simulink model "SMM_1"  (Simulink 8.1)
settings: Solver=ode45  StartTime=0.0  StopTime=20  MaxStep=1e-3  RelTol=1e-4  AbsTol=1e-6
InitFcn:
  | SMM_1_params
values from neighbouring files (symbols this model uses):
  alpha0 = 68  *pi/180    (= 1.18682389136)    [SMM_1_params.m]    (also in SMM_1_returnMap.m; SMM_1_roughTerrain.m)
  dx0 = 5    [SMM_1_params.m]    (also in SMM_1_returnMap.m = sqrt(2/m*(Esys-m*g*y0)))
  dy0 = 0    [SMM_1_params.m]    (also in SMM_1_returnMap.m; SMM_1_roughTerrain.m)
  g = 9.81    [SMM_1_params.m]    (also in SMM_1_returnMap.m; SMM_1_roughTerrain.m)
  k = 20000    [SMM_1_params.m]    (also in SMM_1_returnMap.m; SMM_1_roughTerrain.m)
  l0 = 1    [SMM_1_params.m]    (also in SMM_1_returnMap.m; SMM_1_roughTerrain.m)
  m = 70    [SMM_1_params.m]    (also in SMM_1_returnMap.m; SMM_1_roughTerrain.m)
  x0 = 0    [SMM_1_params.m]    (also in SMM_1_returnMap.m; SMM_1_roughTerrain.m)
  y0 = 1    [SMM_1_params.m]    (also in SMM_1_returnMap.m = v_y0(state))
libraries: simulink x1, simulink_extras x1
settings Model: Creator=hgeyer  LastModifiedBy=benshih
settings DebuggingCC: FcnCallInpInsideContextMsg=EnableAllAsWarning
settings GRTTargetCC: CombineOutputUpdateFcns=on  GRTInterface=off

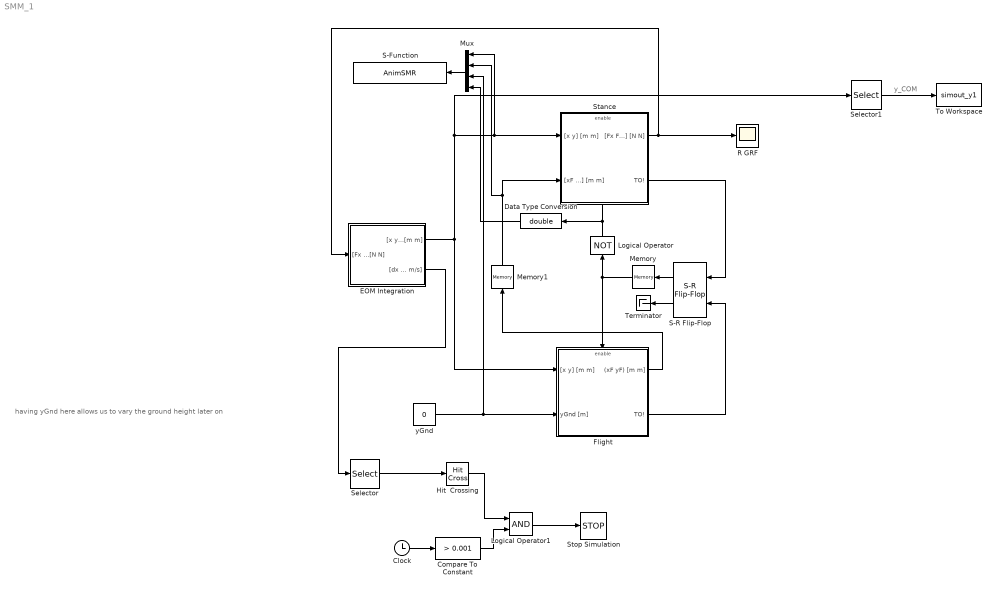
== system SMM_1 ==
  note: y_COM
  note: having yGnd here allows
      | us to vary the ground height later on
  Clock : Clock
  Compare To Constant : simulink/Logic and Bit Operations/Compare To Constant  relop=>  const=0.001  OutDataTypeStr=boolean
  Data Type Conversion : DataTypeConversion  OutDataTypeStr=double
  EOM Integration : Subsystem
  Flight : Subsystem
  Hit  Crossing : HitCross  HitCrossingDirection=falling
  Logical Operator : Logic  Operator=NOT  AllPortsSameDT=off  OutDataTypeStr=boolean
  Logical Operator1 : Logic  AllPortsSameDT=off  OutDataTypeStr=boolean
  Memory : Memory  X0=1
  Memory1 : Memory  X0=[0 0]
  Mux : Mux
  R GRF : Scope
  S-Function : S-Function  FunctionName=AnimSMR  Parameters=0.01  EnableBusSupport=off
  S-R Flip-Flop : simulink_extras/Flip Flops/S-R Flip-Flop  initial_condition=1
  Selector : Selector  InputPortWidth=2  IndexOptions=Index vector (dialog)  Indices=2  OutputSizes=1
  Selector1 : Selector  InputPortWidth=2  IndexOptions=Index vector (dialog)  Indices=2  OutputSizes=1
  Stance : Subsystem
  Stop Simulation : Stop
  Terminator : Terminator
  To Workspace : ToWorkspace  VariableName=simout_y1  SampleTime=-1
      settings: MaxDataPoints=1
  yGnd : Constant  Value=0
  wires:
  EOM Integration/1("[x y] [m m]") -> Flight/1("[x y] [m m]"), Selector1/1, Mux/1, Stance/1("[x y] [m m]")
  Stance/2(TO!) -> S-R Flip-Flop/1
  S-R Flip-Flop/1 -> Memory/1
  Logical Operator/1 -> Stance/Enable, Data Type Conversion/1
  Memory/1 -> Logical Operator/1, Flight/Enable
  Flight/2(TO!) -> S-R Flip-Flop/2
  Flight/1((xF yF) [m m]) -> Memory1/1
  Memory1/1 -> Mux/2, Stance/2("[xF yF] [m m]")
  Mux/1 -> S-Function/1
  S-R Flip-Flop/2 -> Terminator/1
  Stance/1("[Fx Fy] [N N]") -> R GRF/1, EOM Integration/1("[Fx Fy] [N N]")
  yGnd/1 -> Flight/2(yGnd [m]), Mux/3
  Data Type Conversion/1 -> Mux/4
  EOM Integration/2("[dx dy] [m/s m/s]") -> Selector/1
  Selector/1 -> Hit  Crossing/1
  Hit  Crossing/1 -> Logical Operator1/1
  Clock/1 -> Compare To Constant/1
  Compare To Constant/1 -> Logical Operator1/2
  Logical Operator1/1 -> Stop Simulation/1
  Selector1/1 -> To Workspace/1

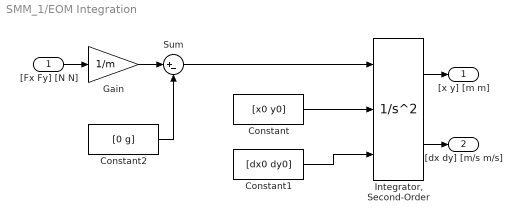
== system SMM_1/EOM Integration ==
  "[Fx Fy] [N N]" : Inport
  Constant : Constant  Value=[x0 y0]
  Constant1 : Constant  Value=[dx0 dy0]
  Constant2 : Constant  Value=[0 g]
  Gain : Gain  Gain=1/m
  "Integrator, Second-Order" : SecondOrderIntegrator  ICSourceX=external  ICSourceDXDT=external
  Sum : Sum  Inputs=|+-
  "[x y] [m m]" : Outport
  "[dx dy] [m/s m/s]" : Outport  Port=2
  wires:
  Constant/1 -> "Integrator, Second-Order"/2
  Constant1/1 -> "Integrator, Second-Order"/3
  Gain/1 -> Sum/1
  Sum/1 -> "Integrator, Second-Order"/1
  Constant2/1 -> Sum/2
  "[Fx Fy] [N N]"/1 -> Gain/1
  "Integrator, Second-Order"/1 -> "[x y] [m m]"/1
  "Integrator, Second-Order"/2 -> "[dx dy] [m/s m/s]"/1

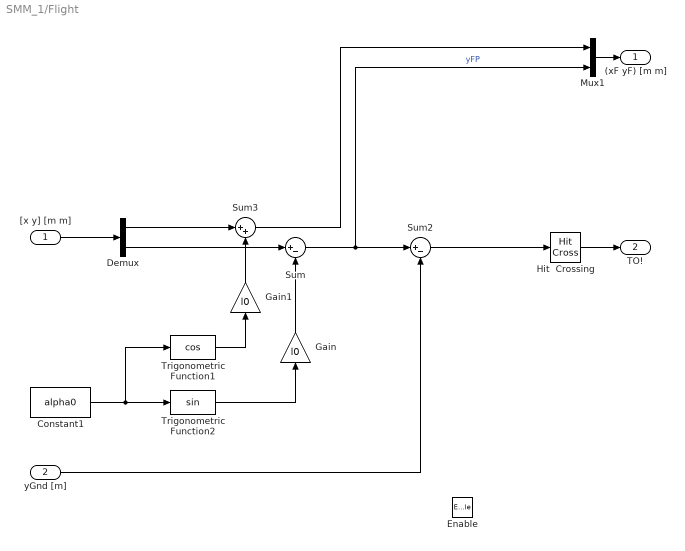
== system SMM_1/Flight ==
  "[x y] [m m]" : Inport
  yGnd [m] : Inport  Port=2
  Enable : EnablePort  StatesWhenEnabling=reset
  Constant1 : Constant  Value=alpha0
  Demux : Demux  Outputs=2
  Gain : Gain  Gain=l0
  Gain1 : Gain  Gain=l0
  Hit  Crossing : HitCross  HitCrossingDirection=falling
  Mux1 : Mux  Inputs=2
  Sum : Sum  Inputs=|+-
  Sum2 : Sum  Inputs=|+-
  Sum3 : Sum  Inputs=|++
  Trigonometric Function1 : Trigonometry  Operator=cos
  Trigonometric Function2 : Trigonometry
  (xF yF) [m m] : Outport  InitialOutput=0
  TO! : Outport  Port=2  OutputWhenDisabled=reset  InitialOutput=0
  wires:
  Hit  Crossing/1 -> TO!/1
  Mux1/1 -> (xF yF) [m m]/1
  "[x y] [m m]"/1 -> Demux/1
  Demux/2 -> Sum/1
  Constant1/1 -> Trigonometric Function2/1, Trigonometric Function1/1
  Trigonometric Function2/1 -> Gain/1
  Gain/1 -> Sum/2
  Sum/1 -> Sum2/1, Mux1/2  "yFP"
  yGnd [m]/1 -> Sum2/2
  Sum2/1 -> Hit  Crossing/1
  Trigonometric Function1/1 -> Gain1/1
  Gain1/1 -> Sum3/2
  Demux/1 -> Sum3/1
  Sum3/1 -> Mux1/1

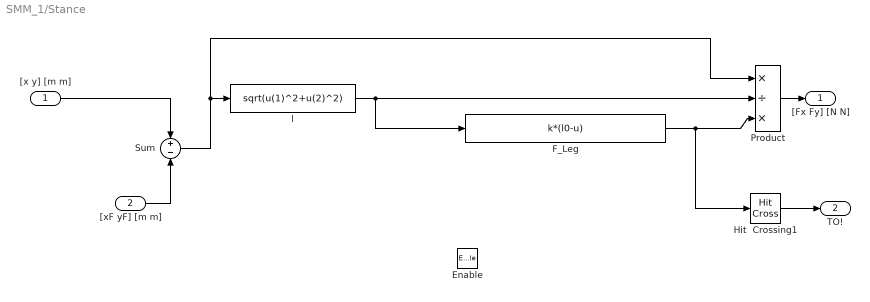
== system SMM_1/Stance ==
  "[x y] [m m]" : Inport
  "[xF yF] [m m]" : Inport  Port=2
  Enable : EnablePort  StatesWhenEnabling=reset
  F_Leg : Fcn  Expr=k*(l0-u)
  Hit  Crossing1 : HitCross  HitCrossingDirection=falling
  Product : Product  Inputs=*/*  RndMeth=Zero
  Sum : Sum  Inputs=+-
  l : Fcn  Expr=sqrt(u(1)^2+u(2)^2)
  "[Fx Fy] [N N]" : Outport  OutputWhenDisabled=reset  InitialOutput=[0 0]
  TO! : Outport  Port=2  OutputWhenDisabled=reset  InitialOutput=0
  wires:
  F_Leg/1 -> Product/3, Hit  Crossing1/1
  l/1 -> Product/2, F_Leg/1
  Product/1 -> "[Fx Fy] [N N]"/1
  "[xF yF] [m m]"/1 -> Sum/2
  "[x y] [m m]"/1 -> Sum/1
  Sum/1 -> l/1, Product/1
  Hit  Crossing1/1 -> TO!/1
